simulink model "MultidifusionEntidades"  (R2023b)
settings: Solver=VariableStepAuto  StartTime=0.0  StopTime=10.0  RelTol=1e-3
undefined symbols (not defined in the file or in its folder): m, n
settings Model: Creator=alfre  LastModifiedBy=alfre

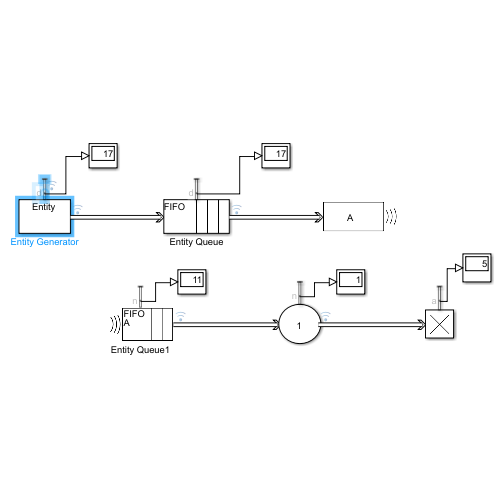
[thumbnail: Simulink's stored preview of the top-level diagram]
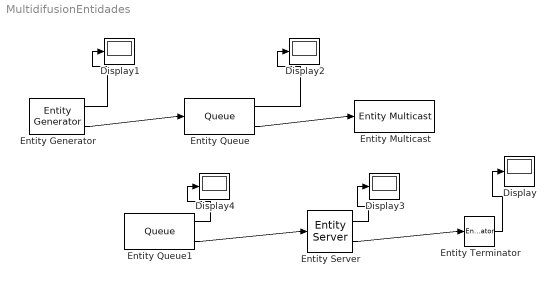
== system MultidifusionEntidades ==
  Display{,1..4} (5 alike) : Display
  Entity Generator : EntityGenerator  OutputPortMessageModes=n,m  TimeSource=MATLAB action  NumberEntitiesDeparted=on  EntityType=Structured  EntityTypeName=Entity
      settings: OutputPortMap=o0,o3
  Entity Multicast : EntityMulticast  Tag=A  InputPortMessageModes=m
  Entity Queue : Queue  InputPortMessageModes=m  OutputPortMessageModes=n,m  NumberEntitiesDeparted=on
      settings: OutputPortMap=o0,o5
  Entity Queue1 : Queue  OutputPortMessageModes=n,m  EntityArrivalSource=Multicast  NumberEntitiesInBlock=on
      settings: OutputPortMap=o1,o5
  Entity Server : EntityServer  InputPortMessageModes=m  OutputPortMessageModes=n,m  Capacity=1  ServiceTimeValue=2  NumberEntitiesInBlock=on
      settings: OutputPortMap=o1,o9
  Entity Terminator : EntityTerminator  InputPortMessageModes=m  NumberEntitiesArrived=on
      settings: OutputPortMap=o0
  wires:
  Entity Generator/2 -> Entity Queue/1
  Entity Queue/2 -> Entity Multicast/1
  Entity Queue1/2 -> Entity Server/1
  Entity Server/2 -> Entity Terminator/1
  Entity Generator/1 -> Display1/1
  Entity Terminator/1 -> Display/1
  Entity Queue/1 -> Display2/1
  Entity Server/1 -> Display3/1
  Entity Queue1/1 -> Display4/1
